simulink model "iterator"  (R2015b)
settings: Solver=FixedStepDiscrete  StartTime=0.0  StopTime=10.0  RelTol=1e-3
settings Model: Creator=d_pal  LastModifiedBy=d_pal

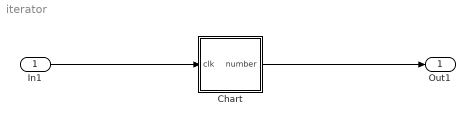
== system iterator ==
  In1 : Inport  SampleTime=0.2
  Chart : Stateflow chart  TreatAsAtomicUnit=on
  Out1 : Outport
  wires:
  In1/1 -> Chart/1(clk)
  Chart/1(number) -> Out1/1

== stateflow chart iterator/Chart ==
  state add
    en: lastInput = clk;
    number = counter;
  (default) -> add
  add -> add : [clk ~= lastInput]
  data: clk input; number output; counter local =0; lastInput local =0
